simulink model "part2alabFP"  (R2014a)
settings: Solver=ode45  StartTime=0.0  StopTime=1.0  FixedStep=0.001  MaxStep=.001  RelTol=1e-3
settings Model: Creator=nandi2  LastModifiedBy=nandi2
settings DataIOCC: LimitDataPoints=off

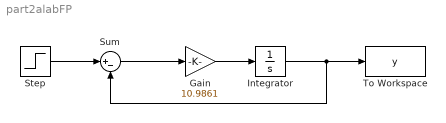
== system part2alabFP ==
  Gain : Gain  Gain=10.9861
  Integrator : Integrator
  Step : Step  Time=0  After=100  SampleTime=0
  Sum : Sum  Inputs=|+-
  To Workspace : ToWorkspace  VariableName=y  SampleTime=-1
  wires:
  Sum/1 -> Gain/1
  Gain/1 -> Integrator/1
  Integrator/1 -> To Workspace/1, Sum/2
  Step/1 -> Sum/1
